simulink model "main_test_all"  (Simulink 6.3)
settings: Solver=ode45  StartTime=0.0  StopTime=6179  RelTol=1e-3
undefined symbols (not defined in the file): A_att_c, B_att_c, C_att_c, D_att_c, ff_on, q_init, q_ref, t_init, t_step
libraries: components_lib x20, simulink x8
settings Model: Creator=krage  LastModifiedBy=mnkr02  ExtModeAutoUpdateStatusClock=off  StrictBusMsg=None
settings DebuggingCC: CheckSSInitialOutputMsg=off

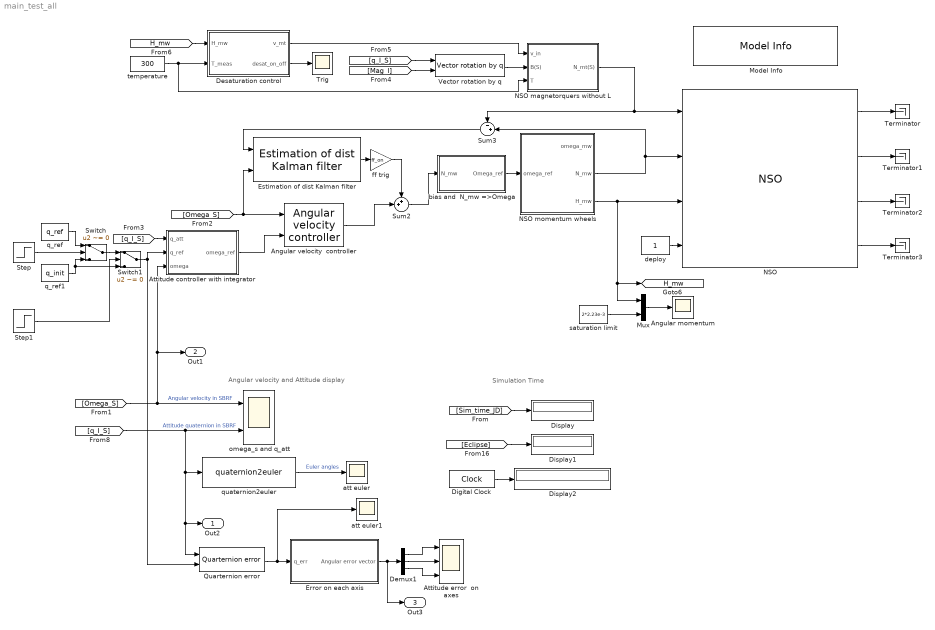
== system main_test_all ==
  note: Simulation Time
  note: Angular velocity and Attitude display
  Angular momentum : Scope
      settings: YMin=0.00125  YMax=0.0045  SaveName=ScopeData2
  Angular velocity  controller : components_lib/ACS/Controllers/Angular velocity  controller  ang_file_name='ang_robust_control.m'
  Attitude controller with integrator : Subsystem  AncestorBlock=components_lib/ACS/Controllers/Attitude controller with integrator  mask(Attitude Controller){att_file_name='att_control_with_integrator.m'}
      mask prompts: att_file_name "Attitude controller design file name (remember gnyfs :-))"
      mask help:
      | The controller in this block is to be constructed using a state space system. The error quarternion is calculated from the input and the result is used in the SS-system. Thus if the controller is merely a gain matrix only the D-matrix has to contain the controller and the remaining be zero-matrices. The controller design files are kept in the "design" directory and the definition of the controller system matrices is the final task in each controller design file.
      | The different matrices for the state space system are named:
      | A_att_c
      | B_att_c
      | C_att_c
      | D_att_c
      mask init:
      | run(strcat('design/',att_file_name))
  Attitude error  on axes : Scope  NumInputPorts=3
      settings: YMin=-3.5~-5~-5  YMax=3.5~5~5  SaveName=ScopeData5
  Demux1 : Demux  Outputs=3
  Desaturation control : Subsystem  mask{h_bias=2.23*1e-3, desat_on=0.7*2.23e-3, desat_off=0.01*2.23e-3}
      mask prompts: h_bias "Angular momentum bias"; desat_on "Threshold desaturation on"; desat_off "Threshold desaturation off"
  Digital Clock : DigitalClock
  Display : Display
  Display1 : Display
  Display2 : Display
  Error on each axis : Subsystem
  Estimation of dist Kalman filter : components_lib/ACS/Controllers/Estimation of dist Kalman filter  ang_file_name='kalman_estimator.m'
  Model Info : simulink/Model-Wide Utilities/Model Info  InitialBlockCM=None  BlockCM=None  Frame=on  DisplayStringWithTags=|  HorizontalTextAlignment=Center  LeftAlignmentValue=0.5  SourceBlockDiagram=main_test_all  TagMaxNumber=20
      | sun to eclipse : 2452315.560376
      | 32 sec. before : 2452315.56
      | eclipse to sun : 2452315.513363
  Mux : Mux  Inputs=2
  NSO : components_lib/NSO  Tag=AAUSAT-II Model  Description=AAUSAT-II Model  r_com_s=[0.05 0.05 0.15]  sat_temp_start=0  r_com_s_deployed=[0.05 0.05 0.125]  mass_sc=3  Dim=[0.1 0.1 0.3]  inertia_c=[25 25 5]/1e3  inertia_d=I_sat  init_jd=2452315.56  q_s_c=[0 0 0 1]  q_init_s_i=q_init  w_init_s=omega_init  Cd=drag_coef  rho=ro_air  enable_sensor_emulation=off  alb_emu_enabled=off  enable_dist=on
  NSO magnetorquers without L : Subsystem  AncestorBlock=components_lib/Actuator Emulation/NSO magnetorquers without L
  NSO momentum wheels : Subsystem  AncestorBlock=components_lib/Actuator Emulation/NSO momentum wheels  mask{w_mw_i=[1078.6 1078.6 1078.6] *0.5}
      mask prompts: w_mw_i "Initial Angular Velocity"
  Quarternion error : components_lib/Math utilities/Quaternion operations/Quarternion error
  Step : Step  Time=t_step  Before=1  After=0  SampleTime=0
  Step1 : Step  Time=t_init  SampleTime=0
  Sum2 : Sum  Inputs=++|
  Sum3 : Sum  Orientation=left  Inputs=-+|
  Switch : Switch  Criteria=u2 ~= 0
  Switch1 : Switch  Criteria=u2 ~= 0
  Terminator{,1..3} (4 alike) : Terminator
  Trig : Scope
      settings: YMin=0.95  YMax=1.05  SaveName=ScopeData3
  Vector rotation by q : components_lib/Math utilities/Quaternion operations/Vector rotation by q
  att euler : Scope
      settings: YMin=-3.5  YMax=3.5
  att euler1 : Scope
      settings: YMin=-3.5  YMax=3.5  SaveName=ScopeData7
  bias and  N_mw =>Omega : Subsystem
  deploy : Constant
  ff trig : Gain  Gain=ff_on
  omega_s and q_att : Scope  NumInputPorts=2
      settings: YMin=-0.4~-1  YMax=0.15~1
  q_ref : Constant  Value=q_ref
  q_ref1 : Constant  Value=q_init
  quaternion2euler : components_lib/Math utilities/Quaternion operations/quaternion2euler
  saturation limit : Constant  Value=2*2.23e-3
  temperature : Constant  Value=300
  Out2 : Outport
  Out1 : Outport  Port=2
  Out3 : Outport  Port=3
  tag scope: H_mw=global
  wires:
  [q_I_S] -> omega_s and q_att/2, quaternion2euler/1, Out2/1, Quarternion error/1  "Attitude quaternion in SBRF"
  quaternion2euler/1 -> att euler/1  "Euler angles"
  [Sim_time_JD] -> Display/1
  [Eclipse] -> Display1/1
  Digital Clock/1 -> Display2/1
  deploy/1 -> NSO/4
  [q_I_S] -> Attitude controller with integrator/1(q_att)
  [Omega_S] -> Angular velocity  controller/1, Estimation of dist Kalman filter/2
  Attitude controller with integrator/1(omega_ref) -> Angular velocity  controller/2
  temperature/1 -> Desaturation control/2(T_meas), NSO magnetorquers without L/3(T)
  [Mag_I] -> Vector rotation by q/2
  [q_I_S] -> Vector rotation by q/1
  Vector rotation by q/1 -> NSO magnetorquers without L/2(B(S))
  Desaturation control/1(v_mt) -> NSO magnetorquers without L/1(v_in)
  [H_mw] -> Desaturation control/1(H_mw)
  NSO magnetorquers without L/1(N_mt(S)) -> NSO/1, Sum3/1
  Desaturation control/2(desat_on_off) -> Trig/1
  NSO momentum wheels/3(H_mw) -> NSO/3, [H_mw], Mux/1
  NSO momentum wheels/2(N_mw) -> NSO/2, Sum3/2
  bias and  N_mw =>Omega/1(Omega_ref) -> NSO momentum wheels/1(omega_ref)
  Mux/1 -> Angular momentum/1
  saturation limit/1 -> Mux/2
  [Omega_S] -> omega_s and q_att/1, Out1/1, Attitude controller with integrator/3(omega)  "Angular velocity in SBRF"
  Angular velocity  controller/1 -> Sum2/2
  Sum2/1 -> bias and  N_mw =>Omega/1(N_mw)
  Sum3/1 -> Estimation of dist Kalman filter/1
  NSO/1 -> Terminator/1
  NSO/2 -> Terminator1/1
  NSO/3 -> Terminator2/1
  NSO/4 -> Terminator3/1
  Estimation of dist Kalman filter/1 -> ff trig/1
  ff trig/1 -> Sum2/1
  Quarternion error/1 -> Error on each axis/1(q_err), att euler1/1
  Error on each axis/1(Angular error vector) -> Demux1/1, Out3/1
  Demux1/1 -> Attitude error  on axes/1
  Demux1/2 -> Attitude error  on axes/2
  Demux1/3 -> Attitude error  on axes/3
  q_ref1/1 -> Switch/3, Switch1/3
  q_ref/1 -> Switch/1
  Step/1 -> Switch/2
  Switch/1 -> Switch1/1
  Switch1/1 -> Attitude controller with integrator/2(q_ref), Quarternion error/2
  Step1/1 -> Switch1/2

== system main_test_all/Attitude controller with integrator ==
  q_att : Inport
  q_ref : Inport  Port=2
  omega : Inport  Port=3
  Integrator : Integrator  LimitOutput=on  UpperSaturationLimit=0.01  LowerSaturationLimit=-0.01
  Mux : Mux  Inputs=3
  Quarternion error : components_lib/Math utilities/Quaternion operations/Quarternion error
  Scope : Scope
      settings: SaveName=ScopeData10
  Selector : Selector  Elements=[1 2 3]  InputPortWidth=4
  State-Space : StateSpace  A=A_att_c  B=B_att_c  C=C_att_c  D=D_att_c
  omega_ref : Outport
  wires:
  Integrator/1 -> Mux/3, Scope/1
  State-Space/1 -> omega_ref/1
  Quarternion error/1 -> Selector/1
  q_att/1 -> Quarternion error/1
  q_ref/1 -> Quarternion error/2
  Selector/1 -> Integrator/1, Mux/1
  omega/1 -> Mux/2
  Mux/1 -> State-Space/1

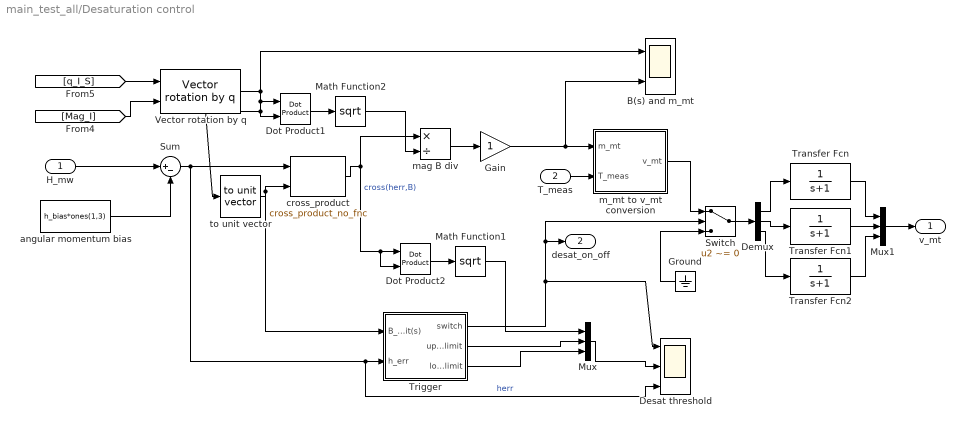
== system main_test_all/Desaturation control ==
  H_mw : Inport
  T_meas : Inport  Port=2
  B(s) and m_mt : Scope  NumInputPorts=2
      settings: YMin=-2e-005~-1  YMax=2e-005~11  SaveName=ScopeData6
  Demux : Demux  Outputs=3
  Desat threshold : Scope  NumInputPorts=3
      settings: YMin=0~0~-0.0025  YMax=1~0.004~0.0025  SaveName=desat_info
  Dot Product1 : simulink/Math Operations/Dot Product  InputSameDT=on  OutDataType=sfix(16)  OutScaling=2^-10  DoSatur=off
  Dot Product2 : simulink/Math Operations/Dot Product  InputSameDT=on  OutDataType=sfix(16)  OutScaling=2^-10  DoSatur=off
  Gain : Gain
  Ground : Ground  Orientation=left
  Math Function1 : Math  Operator=sqrt  SaturateOnIntegerOverflow=on
  Math Function2 : Math  Operator=sqrt  SaturateOnIntegerOverflow=on
  Mux : Mux  Inputs=3
  Mux1 : Mux  Inputs=3
  Sum : Sum  Inputs=|+-
  Switch : Switch  Criteria=u2 ~= 0  Threshold=0.5
  Transfer Fcn : TransferFcn  Denominator=[1 1]
  Transfer Fcn1 : TransferFcn  Denominator=[1 1]
  Transfer Fcn2 : TransferFcn  Denominator=[1 1]
  Trigger : Subsystem
  Vector rotation by q : components_lib/Math utilities/Quaternion operations/Vector rotation by q
  angular momentum bias : Constant  Value=h_bias*ones(1,3)
  cross_product : components_lib/Math utilities/Vector operations/cross_product_no_fnc
  m_mt to v_mt conversion : Subsystem  mask{n_mt=[435 435 865], A_mt=[0.21*0.07 0.21*0.07 0.07*0.07], L_mt=[26.956e-3 26.956e-3 59.256e-3], v_max_mt=5}
      mask prompts: n_mt "Coil winding number [n_x n_y n_z]"; A_mt "Coil area [A_mt_x A_mt_y A_mt_z]"; L_mt "Coil inductance [L_mt_x L_mt_y L_mt_z]"; v_max_mt "Maximum voltage"
  mag B div : Product  Inputs=*/  OutScaling=2^-10
  to unit vector : components_lib/Math utilities/Vector operations/to unit vector
  v_mt : Outport
  desat_on_off : Outport  Port=2
  wires:
  H_mw/1 -> Sum/1
  angular momentum bias/1 -> Sum/2
  [Mag_I] -> Vector rotation by q/2
  [q_I_S] -> Vector rotation by q/1
  Sum/1 -> cross_product/1, Trigger/2(h_err), Desat threshold/3  "herr"
  Vector rotation by q/1 -> Dot Product1/1, Dot Product1/2, to unit vector/1, B(s) and m_mt/1
  cross_product/1 -> mag B div/1, Dot Product2/1, Dot Product2/2  "cross(herr,B)"
  Ground/1 -> Switch/3
  T_meas/1 -> m_mt to v_mt conversion/2(T_meas)
  mag B div/1 -> Gain/1
  m_mt to v_mt conversion/1(v_mt) -> Switch/1
  Dot Product1/1 -> Math Function2/1
  Math Function2/1 -> mag B div/2
  Gain/1 -> m_mt to v_mt conversion/1(m_mt), B(s) and m_mt/2
  to unit vector/1 -> cross_product/2, Trigger/1(B_unit(s))
  Switch/1 -> Demux/1
  Demux/1 -> Transfer Fcn/1
  Demux/2 -> Transfer Fcn1/1
  Demux/3 -> Transfer Fcn2/1
  Transfer Fcn/1 -> Mux1/1
  Transfer Fcn1/1 -> Mux1/2
  Transfer Fcn2/1 -> Mux1/3
  Mux1/1 -> v_mt/1
  Mux/1 -> Desat threshold/2
  Trigger/1(switch) -> Desat threshold/1, desat_on_off/1, Switch/2
  Trigger/2(upper limit) -> Mux/2
  Dot Product2/1 -> Math Function1/1
  Math Function1/1 -> Mux/1
  Trigger/3(lower limit) -> Mux/3

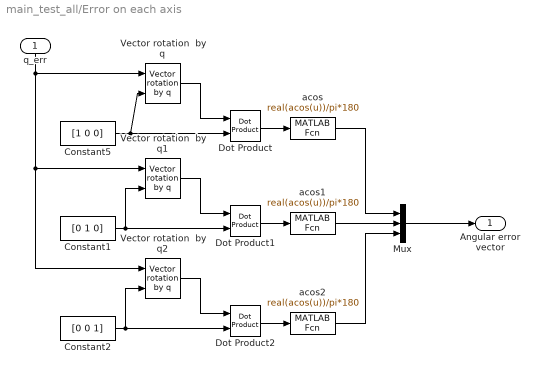
== system main_test_all/Error on each axis ==
  q_err : Inport  Orientation=down
  Constant1 : Constant  Value=[0 1 0]
  Constant2 : Constant  Value=[0 0 1]
  Constant5 : Constant  Value=[1 0 0]
  Dot Product : simulink/Math Operations/Dot Product  InputSameDT=on  OutDataType=sfix(16)  OutScaling=2^-10  DoSatur=off
  Dot Product1 : simulink/Math Operations/Dot Product  InputSameDT=on  OutDataType=sfix(16)  OutScaling=2^-10  DoSatur=off
  Dot Product2 : simulink/Math Operations/Dot Product  InputSameDT=on  OutDataType=sfix(16)  OutScaling=2^-10  DoSatur=off
  Mux : Mux  Inputs=3
  Vector rotation  by q : components_lib/Math utilities/Quaternion operations/Vector rotation by q
  Vector rotation  by q1 : components_lib/Math utilities/Quaternion operations/Vector rotation by q
  Vector rotation  by q2 : components_lib/Math utilities/Quaternion operations/Vector rotation by q
  acos : MATLABFcn  MATLABFcn=real(acos(u))/pi*180
  acos1 : MATLABFcn  MATLABFcn=real(acos(u))/pi*180
  acos2 : MATLABFcn  MATLABFcn=real(acos(u))/pi*180
  Angular error vector : Outport
  wires:
  Constant5/1 -> Dot Product/2, Vector rotation  by q/2
  Vector rotation  by q/1 -> Dot Product/1
  Dot Product/1 -> acos/1
  q_err/1 -> Vector rotation  by q/1, Vector rotation  by q1/1, Vector rotation  by q2/1
  Constant1/1 -> Vector rotation  by q1/2, Dot Product1/2
  Vector rotation  by q1/1 -> Dot Product1/1
  Dot Product1/1 -> acos1/1
  Constant2/1 -> Vector rotation  by q2/2, Dot Product2/2
  Vector rotation  by q2/1 -> Dot Product2/1
  Dot Product2/1 -> acos2/1
  acos/1 -> Mux/1
  acos1/1 -> Mux/2
  acos2/1 -> Mux/3
  Mux/1 -> Angular error vector/1

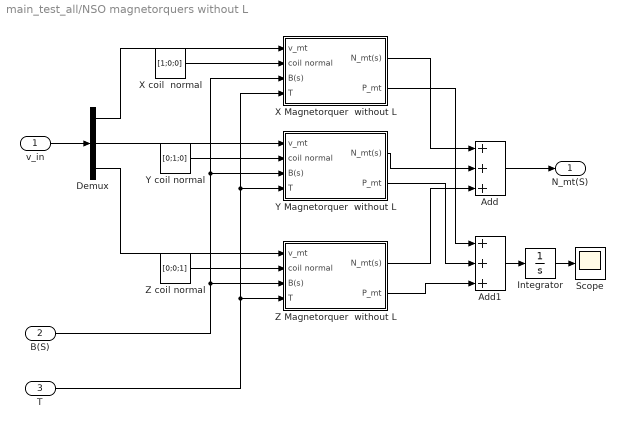
== system main_test_all/NSO magnetorquers without L ==
  v_in : Inport
  B(S) : Inport  Port=2
  T : Inport  Port=3
  Add : Sum  Inputs=+++  OutScaling=2^-10
  Add1 : Sum  Inputs=+++  OutScaling=2^-10
  Demux : Demux  Outputs=3
  Integrator : Integrator
  Scope : Scope
      settings: YMin=24.35  YMax=25.2  SaveName=power_mt
  "X Magnetorquer  without L " : Subsystem  AncestorBlock=components_lib/Actuator Emulation/Magnetorquer without L  mask{v_max_mt=5, coil_dim=[0.07 0.21], n_mt=435, A_wire_mt=(pi/4)*0.0002^2, sigma_0_mt=1.7e-8, alpha_0_mt=3.9e-3, T_0_mt=293}
      mask prompts: v_max_mt "Maximum voltage"; coil_dim "Coil dimensions [x y]"; n_mt "Coil winding number"; A_wire_mt "Wire cross sectional area"; sigma_0_mt "Wire resistivity"; alpha_0_mt "Wire resistivity temp. coef."; T_0_mt "Wire resistivity base temp."
  X coil  normal : Constant  Value=[1;0;0]
  Y Magnetorquer  without L : Subsystem  AncestorBlock=components_lib/Actuator Emulation/Magnetorquer without L  mask{v_max_mt=5, coil_dim=[0.07 0.21], n_mt=435, A_wire_mt=(pi/4)*0.0002^2, sigma_0_mt=1.7e-8, alpha_0_mt=3.9e-3, T_0_mt=293}
      mask prompts: v_max_mt "Maximum voltage"; coil_dim "Coil dimensions [x y]"; n_mt "Coil winding number"; A_wire_mt "Wire cross sectional area"; sigma_0_mt "Wire resistivity"; alpha_0_mt "Wire resistivity temp. coef."; T_0_mt "Wire resistivity base temp."
  Y coil normal : Constant  Value=[0;1;0]
  Z Magnetorquer  without L : Subsystem  AncestorBlock=components_lib/Actuator Emulation/Magnetorquer without L  mask{v_max_mt=5, coil_dim=[0.07 0.07], n_mt=865, A_wire_mt=(pi/4)*0.0002^2, sigma_0_mt=1.7e-8, alpha_0_mt=3.9e-3, T_0_mt=293}
      mask prompts: v_max_mt "Maximum voltage"; coil_dim "Coil dimensions [x y]"; n_mt "Coil winding number"; A_wire_mt "Wire cross sectional area"; sigma_0_mt "Wire resistivity"; alpha_0_mt "Wire resistivity temp. coef."; T_0_mt "Wire resistivity base temp."
  Z coil normal : Constant  Value=[0;0;1]
  N_mt(S) : Outport  PortDimensions=3
  wires:
  v_in/1 -> Demux/1
  Add/1 -> N_mt(S)/1
  X coil  normal/1 -> "X Magnetorquer  without L "/2(coil normal)
  Demux/1 -> "X Magnetorquer  without L "/1(v_mt)
  "X Magnetorquer  without L "/1(N_mt(s)) -> Add/1
  Y Magnetorquer  without L/1(N_mt(s)) -> Add/2
  Z Magnetorquer  without L/1(N_mt(s)) -> Add/3
  Demux/2 -> Y Magnetorquer  without L/1(v_mt)
  Y coil normal/1 -> Y Magnetorquer  without L/2(coil normal)
  Demux/3 -> Z Magnetorquer  without L/1(v_mt)
  Z coil normal/1 -> Z Magnetorquer  without L/2(coil normal)
  B(S)/1 -> Z Magnetorquer  without L/3(B(s)), Y Magnetorquer  without L/3(B(s)), "X Magnetorquer  without L "/3(B(s))
  T/1 -> Z Magnetorquer  without L/4(T), Y Magnetorquer  without L/4(T), "X Magnetorquer  without L "/4(T)
  "X Magnetorquer  without L "/2(P_mt) -> Add1/1
  Y Magnetorquer  without L/2(P_mt) -> Add1/2
  Z Magnetorquer  without L/2(P_mt) -> Add1/3
  Add1/1 -> Integrator/1
  Integrator/1 -> Scope/1

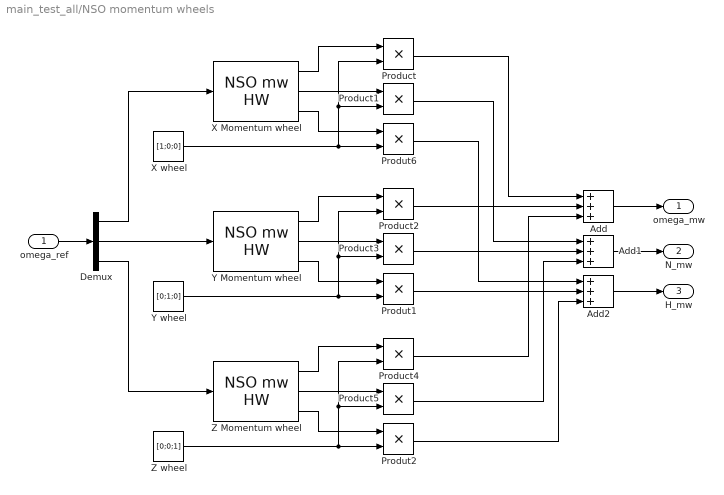
== system main_test_all/NSO momentum wheels ==
  omega_ref : Inport
  Add : Sum  Inputs=+++  OutScaling=2^-10
  Add1 : Sum  Inputs=+++  OutScaling=2^-10
  Add2 : Sum  Inputs=+++  OutScaling=2^-10
  Demux : Demux  Outputs=3
  Product{,1..5} (6 alike) : Product  RndMeth=Zero
  Produt1 : Product  RndMeth=Zero
  Produt2 : Product  RndMeth=Zero
  Produt6 : Product  RndMeth=Zero
  X Momentum wheel : components_lib/Actuator Emulation/NSO mw HW  C_p=0.01  C_i=0.001  w_mw_init=w_mw_i(1)
  X wheel : Constant  Value=[1;0;0]
  Y Momentum wheel : components_lib/Actuator Emulation/NSO mw HW  C_p=0.01  C_i=0.001  w_mw_init=w_mw_i(2)
  Y wheel : Constant  Value=[0;1;0]
  Z Momentum wheel : components_lib/Actuator Emulation/NSO mw HW  C_p=0.01  C_i=0.001  w_mw_init=w_mw_i(3)
  Z wheel : Constant  Value=[0;0;1]
  omega_mw : Outport  PortDimensions=3
  N_mw : Outport  Port=2  PortDimensions=3
  H_mw : Outport  Port=3  PortDimensions=3
  wires:
  Demux/2 -> Y Momentum wheel/1
  Demux/3 -> Z Momentum wheel/1
  Demux/1 -> X Momentum wheel/1
  omega_ref/1 -> Demux/1
  Product4/1 -> Add/3
  Product5/1 -> Add1/3
  Produt2/1 -> Add2/3
  Z Momentum wheel/2 -> Product5/1
  Z Momentum wheel/1 -> Product4/1
  Z Momentum wheel/3 -> Produt2/1
  Z wheel/1 -> Produt2/2, Product5/2, Product4/2
  Produt1/1 -> Add2/2
  Product3/1 -> Add1/2
  Product2/1 -> Add/2
  Y Momentum wheel/2 -> Product3/1
  Y Momentum wheel/1 -> Product2/1
  Y Momentum wheel/3 -> Produt1/1
  Y wheel/1 -> Produt1/2, Product3/2, Product2/2
  X Momentum wheel/2 -> Product1/1
  X Momentum wheel/1 -> Product/1
  X Momentum wheel/3 -> Produt6/1
  Add/1 -> omega_mw/1
  X wheel/1 -> Produt6/2, Product1/2, Product/2
  Add1/1 -> N_mw/1
  Product/1 -> Add/1
  Product1/1 -> Add1/1
  Add2/1 -> H_mw/1
  Produt6/1 -> Add2/1

== system main_test_all/bias and  N_mw =>Omega ==
  N_mw : Inport
  I_FW : Gain  Gain=1/4.139e-6
  Integrator : Integrator  InitialCondition=[2.23 2.23 2.23]*1e-3
  Sum : Sum  Inputs=|++
  angular velocity bias : Constant  Value=[1078.6 1078.6 1078.6] *0.5
  Omega_ref : Outport
  wires:
  I_FW/1 -> Sum/1
  angular velocity bias/1 -> Sum/2
  Integrator/1 -> I_FW/1
  N_mw/1 -> Integrator/1
  Sum/1 -> Omega_ref/1

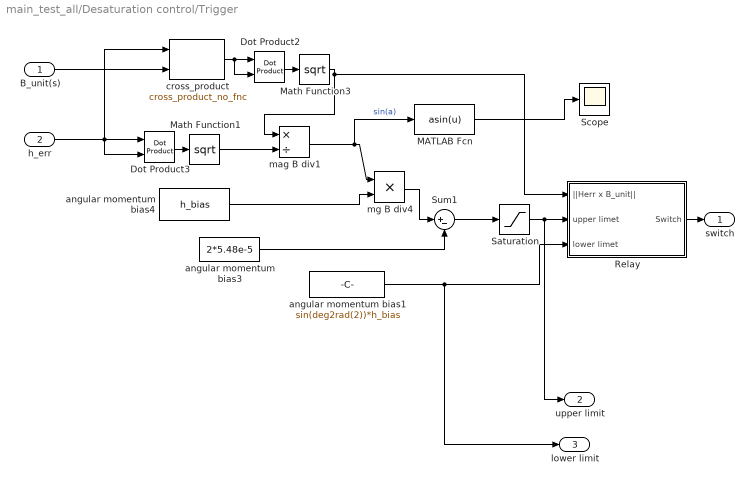
== system main_test_all/Desaturation control/Trigger ==
  B_unit(s) : Inport  PortDimensions=3
  h_err : Inport  Port=2
  Dot Product2 : simulink/Math Operations/Dot Product  InputSameDT=on  OutDataType=sfix(16)  OutScaling=2^-10  DoSatur=off
  Dot Product3 : simulink/Math Operations/Dot Product  InputSameDT=on  OutDataType=sfix(16)  OutScaling=2^-10  DoSatur=off
  MATLAB Fcn : MATLABFcn  MATLABFcn=asin(u)
  Math Function1 : Math  Operator=sqrt  SaturateOnIntegerOverflow=on
  Math Function3 : Math  Operator=sqrt  SaturateOnIntegerOverflow=on
  Relay : Subsystem
  Saturation : Saturate  UpperLimit=inf  LowerLimit=2*sin(deg2rad(2))*h_bias
  Scope : Scope
      settings: YMin=0.5  YMax=1.6  SaveName=ScopeData4
  Sum1 : Sum  Inputs=|+-
  angular momentum bias1 : Constant  Value=sin(deg2rad(2))*h_bias
  angular momentum bias3 : Constant  Value=2*5.48e-5
  angular momentum bias4 : Constant  Value=h_bias
  cross_product : components_lib/Math utilities/Vector operations/cross_product_no_fnc
  mag B div1 : Product  Inputs=*/  OutScaling=2^-10
  mg B div4 : Product  OutScaling=2^-10
  switch : Outport
  upper limit : Outport  Port=2
  lower limit : Outport  Port=3
  wires:
  angular momentum bias3/1 -> Sum1/2
  Relay/1(Switch) -> switch/1
  angular momentum bias4/1 -> mg B div4/2
  mg B div4/1 -> Sum1/1
  Dot Product2/1 -> Math Function3/1
  Dot Product3/1 -> Math Function1/1
  Math Function1/1 -> mag B div1/2
  Sum1/1 -> Saturation/1
  mag B div1/1 -> mg B div4/1, MATLAB Fcn/1  "sin(a)"
  h_err/1 -> Dot Product3/1, Dot Product3/2, cross_product/1
  B_unit(s)/1 -> cross_product/2
  cross_product/1 -> Dot Product2/1, Dot Product2/2
  Math Function3/1 -> mag B div1/1, Relay/1(||Herr x B_unit||)
  angular momentum bias1/1 -> Relay/3(lower limet), lower limit/1
  MATLAB Fcn/1 -> Scope/1
  Saturation/1 -> Relay/2(upper limet), upper limit/1

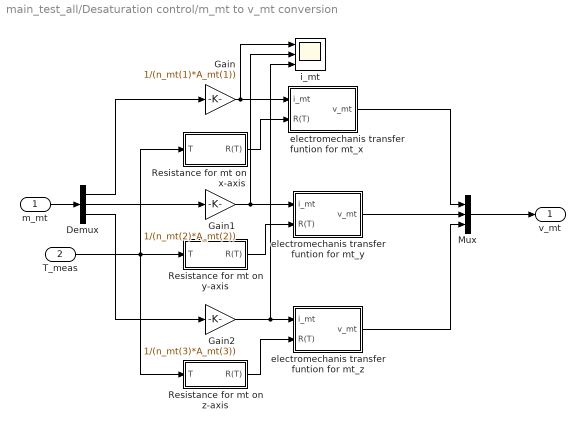
== system main_test_all/Desaturation control/m_mt to v_mt conversion ==
  m_mt : Inport
  T_meas : Inport  Port=2
  Demux : Demux  Outputs=3
  Gain : Gain  Gain=1/(n_mt(1)*A_mt(1))
  Gain1 : Gain  Gain=1/(n_mt(2)*A_mt(2))
  Gain2 : Gain  Gain=1/(n_mt(3)*A_mt(3))
  Mux : Mux  Inputs=3
  Resistance for mt on x-axis : Subsystem  mask{A_wire_mt=(pi/4)*0.0002^2, sigma_0_mt=1.7e-8, alpha_0_mt=3.9e-3, T_0_mt=293}
      mask prompts: A_wire_mt "Wire cross sectional area"; sigma_0_mt "Wire resistivity"; alpha_0_mt "Wire resistivity temp. coef."; T_0_mt "Wire resistivity base temp."
  Resistance for mt on y-axis : Subsystem  mask{A_wire_mt=(pi/4)*0.0002^2, sigma_0_mt=1.7e-8, alpha_0_mt=3.9e-3, T_0_mt=293}
      mask prompts: A_wire_mt "Wire cross sectional area"; sigma_0_mt "Wire resistivity"; alpha_0_mt "Wire resistivity temp. coef."; T_0_mt "Wire resistivity base temp."
  Resistance for mt on z-axis : Subsystem  mask{A_wire_mt=(pi/4)*0.0002^2, sigma_0_mt=1.7e-8, alpha_0_mt=3.9e-3, T_0_mt=293}
      mask prompts: A_wire_mt "Wire cross sectional area"; sigma_0_mt "Wire resistivity"; alpha_0_mt "Wire resistivity temp. coef."; T_0_mt "Wire resistivity base temp."
  electromechanis transfer funtion for mt_x : Subsystem
  "electromechanis transfer funtion for mt_y " : Subsystem
  "electromechanis transfer funtion for mt_z " : Subsystem
  i_mt : Scope  NumInputPorts=3
      settings: YMin=-5~-5~-5  YMax=5~5~5  SaveName=ScopeData8
  v_mt : Outport
  wires:
  Demux/3 -> Gain2/1
  Demux/2 -> Gain1/1
  Demux/1 -> Gain/1
  Gain/1 -> electromechanis transfer funtion for mt_x/1(i_mt), i_mt/1
  Gain1/1 -> "electromechanis transfer funtion for mt_y "/1(i_mt), i_mt/2
  Gain2/1 -> "electromechanis transfer funtion for mt_z "/1(i_mt), i_mt/3
  m_mt/1 -> Demux/1
  "electromechanis transfer funtion for mt_y "/1(v_mt) -> Mux/2
  "electromechanis transfer funtion for mt_z "/1(v_mt) -> Mux/3
  Resistance for mt on x-axis/1(R(T)) -> electromechanis transfer funtion for mt_x/2(R(T))
  Resistance for mt on y-axis/1(R(T)) -> "electromechanis transfer funtion for mt_y "/2(R(T))
  Resistance for mt on z-axis/1(R(T)) -> "electromechanis transfer funtion for mt_z "/2(R(T))
  T_meas/1 -> Resistance for mt on y-axis/1(T), Resistance for mt on x-axis/1(T), Resistance for mt on z-axis/1(T)
  electromechanis transfer funtion for mt_x/1(v_mt) -> Mux/1
  Mux/1 -> v_mt/1

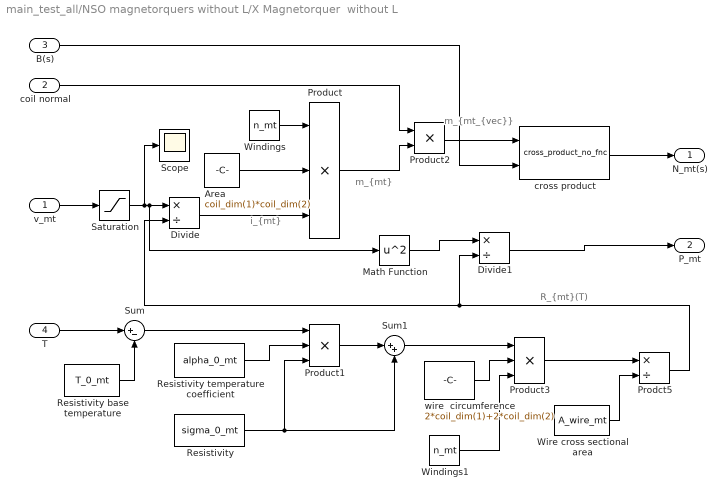
== system main_test_all/NSO magnetorquers without L/X Magnetorquer  without L  ==
  note: R_{mt}(T)
  note: i_{mt}
  note: m_{mt}
  note: m_{mt_{vec}}
  v_mt : Inport
  coil normal : Inport  Port=2
  B(s) : Inport  Port=3
  T : Inport  Port=4
  Area : Constant  Value=coil_dim(1)*coil_dim(2)
  Divide : Product  Inputs=*/  OutScaling=2^-10
  Divide1 : Product  Inputs=*/  OutScaling=2^-10
  Math Function : Math  Operator=square  SaturateOnIntegerOverflow=on
  Prodct5 : Product  Inputs=*/  RndMeth=Zero
  Product : Product  Inputs=3  RndMeth=Zero
  Product1 : Product  Inputs=3  RndMeth=Zero
  Product2 : Product  RndMeth=Zero
  Product3 : Product  Inputs=3  RndMeth=Zero
  Resistivity : Constant  Value=sigma_0_mt
  Resistivity base temperature : Constant  Value=T_0_mt
  Resistivity temperature coefficient : Constant  Value=alpha_0_mt
  Saturation : Saturate  UpperLimit=v_max_mt  LowerLimit=-v_max_mt
  Scope : Scope
      settings: SaveName=ScopeData12
  Sum : Sum  Inputs=|+-
  Sum1 : Sum  Inputs=|++
  Windings : Constant  Value=n_mt
  Windings1 : Constant  Value=n_mt
  Wire cross sectional area : Constant  Value=A_wire_mt
  cross product : components_lib/Math utilities/Vector operations/cross_product_no_fnc
  wire  circumference : Constant  Value=2*coil_dim(1)+2*coil_dim(2)
  N_mt(s) : Outport
  P_mt : Outport  Port=2
  wires:
  Prodct5/1 -> Divide/2, Divide1/2
  Wire cross sectional area/1 -> Prodct5/2
  Product3/1 -> Prodct5/1
  Windings1/1 -> Product3/3
  wire  circumference/1 -> Product3/2
  Sum1/1 -> Product3/1
  Product1/1 -> Sum1/1
  Resistivity/1 -> Sum1/2, Product1/3
  Sum/1 -> Product1/1
  Resistivity temperature coefficient/1 -> Product1/2
  T/1 -> Sum/1
  Resistivity base temperature/1 -> Sum/2
  coil normal/1 -> Product2/1
  v_mt/1 -> Saturation/1
  Saturation/1 -> Divide/1, Math Function/1, Scope/1
  Divide/1 -> Product/3
  Windings/1 -> Product/1
  Area/1 -> Product/2
  Product/1 -> Product2/2
  Product2/1 -> cross product/1
  cross product/1 -> N_mt(s)/1
  B(s)/1 -> cross product/2
  Math Function/1 -> Divide1/1
  Divide1/1 -> P_mt/1

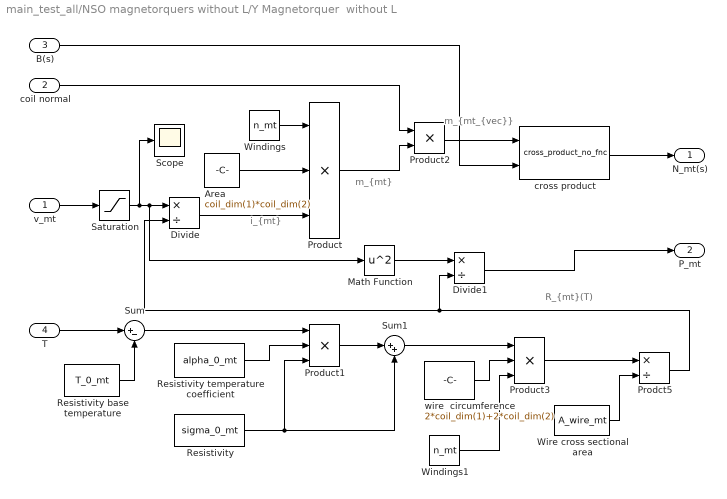
== system main_test_all/NSO magnetorquers without L/Y Magnetorquer  without L ==
  note: R_{mt}(T)
  note: i_{mt}
  note: m_{mt}
  note: m_{mt_{vec}}
  v_mt : Inport
  coil normal : Inport  Port=2
  B(s) : Inport  Port=3
  T : Inport  Port=4
  Area : Constant  Value=coil_dim(1)*coil_dim(2)
  Divide : Product  Inputs=*/  OutScaling=2^-10
  Divide1 : Product  Inputs=*/  OutScaling=2^-10
  Math Function : Math  Operator=square  SaturateOnIntegerOverflow=on
  Prodct5 : Product  Inputs=*/  RndMeth=Zero
  Product : Product  Inputs=3  RndMeth=Zero
  Product1 : Product  Inputs=3  RndMeth=Zero
  Product2 : Product  RndMeth=Zero
  Product3 : Product  Inputs=3  RndMeth=Zero
  Resistivity : Constant  Value=sigma_0_mt
  Resistivity base temperature : Constant  Value=T_0_mt
  Resistivity temperature coefficient : Constant  Value=alpha_0_mt
  Saturation : Saturate  UpperLimit=v_max_mt  LowerLimit=-v_max_mt
  Scope : Scope
      settings: SaveName=ScopeData13
  Sum : Sum  Inputs=|+-
  Sum1 : Sum  Inputs=|++
  Windings : Constant  Value=n_mt
  Windings1 : Constant  Value=n_mt
  Wire cross sectional area : Constant  Value=A_wire_mt
  cross product : components_lib/Math utilities/Vector operations/cross_product_no_fnc
  wire  circumference : Constant  Value=2*coil_dim(1)+2*coil_dim(2)
  N_mt(s) : Outport
  P_mt : Outport  Port=2
  wires:
  Prodct5/1 -> Divide/2, Divide1/2
  Wire cross sectional area/1 -> Prodct5/2
  Product3/1 -> Prodct5/1
  Windings1/1 -> Product3/3
  wire  circumference/1 -> Product3/2
  Sum1/1 -> Product3/1
  Product1/1 -> Sum1/1
  Resistivity/1 -> Sum1/2, Product1/3
  Sum/1 -> Product1/1
  Resistivity temperature coefficient/1 -> Product1/2
  T/1 -> Sum/1
  Resistivity base temperature/1 -> Sum/2
  coil normal/1 -> Product2/1
  v_mt/1 -> Saturation/1
  Saturation/1 -> Divide/1, Math Function/1, Scope/1
  Divide/1 -> Product/3
  Windings/1 -> Product/1
  Area/1 -> Product/2
  Product/1 -> Product2/2
  Product2/1 -> cross product/1
  cross product/1 -> N_mt(s)/1
  B(s)/1 -> cross product/2
  Math Function/1 -> Divide1/1
  Divide1/1 -> P_mt/1

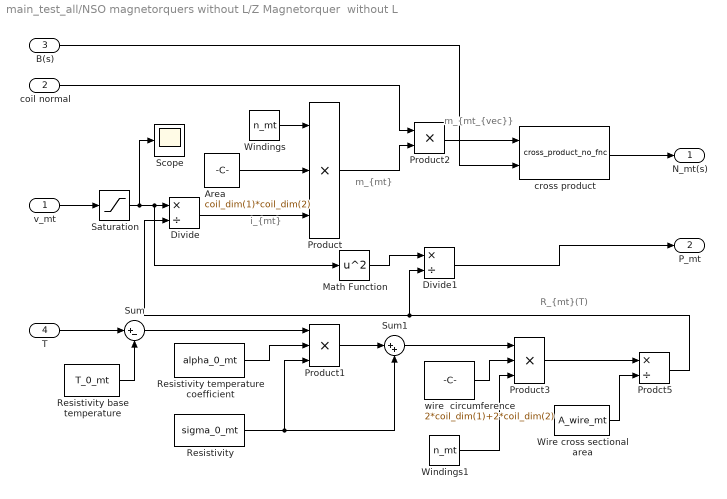
== system main_test_all/NSO magnetorquers without L/Z Magnetorquer  without L ==
  note: R_{mt}(T)
  note: i_{mt}
  note: m_{mt}
  note: m_{mt_{vec}}
  v_mt : Inport
  coil normal : Inport  Port=2
  B(s) : Inport  Port=3
  T : Inport  Port=4
  Area : Constant  Value=coil_dim(1)*coil_dim(2)
  Divide : Product  Inputs=*/  OutScaling=2^-10
  Divide1 : Product  Inputs=*/  OutScaling=2^-10
  Math Function : Math  Operator=square  SaturateOnIntegerOverflow=on
  Prodct5 : Product  Inputs=*/  RndMeth=Zero
  Product : Product  Inputs=3  RndMeth=Zero
  Product1 : Product  Inputs=3  RndMeth=Zero
  Product2 : Product  RndMeth=Zero
  Product3 : Product  Inputs=3  RndMeth=Zero
  Resistivity : Constant  Value=sigma_0_mt
  Resistivity base temperature : Constant  Value=T_0_mt
  Resistivity temperature coefficient : Constant  Value=alpha_0_mt
  Saturation : Saturate  UpperLimit=v_max_mt  LowerLimit=-v_max_mt
  Scope : Scope
      settings: YMin=-1.5  SaveName=ScopeData14
  Sum : Sum  Inputs=|+-
  Sum1 : Sum  Inputs=|++
  Windings : Constant  Value=n_mt
  Windings1 : Constant  Value=n_mt
  Wire cross sectional area : Constant  Value=A_wire_mt
  cross product : components_lib/Math utilities/Vector operations/cross_product_no_fnc
  wire  circumference : Constant  Value=2*coil_dim(1)+2*coil_dim(2)
  N_mt(s) : Outport
  P_mt : Outport  Port=2
  wires:
  Prodct5/1 -> Divide/2, Divide1/2
  Wire cross sectional area/1 -> Prodct5/2
  Product3/1 -> Prodct5/1
  Windings1/1 -> Product3/3
  wire  circumference/1 -> Product3/2
  Sum1/1 -> Product3/1
  Product1/1 -> Sum1/1
  Resistivity/1 -> Sum1/2, Product1/3
  Sum/1 -> Product1/1
  Resistivity temperature coefficient/1 -> Product1/2
  T/1 -> Sum/1
  Resistivity base temperature/1 -> Sum/2
  coil normal/1 -> Product2/1
  v_mt/1 -> Saturation/1
  Saturation/1 -> Divide/1, Math Function/1, Scope/1
  Divide/1 -> Product/3
  Windings/1 -> Product/1
  Area/1 -> Product/2
  Product/1 -> Product2/2
  Product2/1 -> cross product/1
  cross product/1 -> N_mt(s)/1
  B(s)/1 -> cross product/2
  Math Function/1 -> Divide1/1
  Divide1/1 -> P_mt/1

== system main_test_all/Desaturation control/Trigger/Relay ==
  ||Herr x B_unit|| : Inport  Orientation=down
  upper limet : Inport  Port=2
  lower limet : Inport  Port=3
  Logical Operator1 : Logic  AllPortsSameDT=off  OutDataTypeMode=Boolean
  Logical Operator2 : Logic  Operator=OR  AllPortsSameDT=off  OutDataTypeMode=Boolean
  Logical Operator3 : Logic  AllPortsSameDT=off  OutDataTypeMode=Boolean
  Memory : Memory  Orientation=left
  Relational Operator : RelationalOperator  Operator=>  LogicOutDataTypeMode=Boolean  LogicDataType=1
  Relational Operator1 : RelationalOperator  Operator=>  LogicOutDataTypeMode=Boolean  LogicDataType=1
  Switch : Outport
  wires:
  ||Herr x B_unit||/1 -> Relational Operator/1, Relational Operator1/1
  Relational Operator1/1 -> Logical Operator1/1, Logical Operator3/2
  Logical Operator1/1 -> Logical Operator2/2
  Logical Operator2/1 -> Memory/1, Switch/1
  Memory/1 -> Logical Operator1/2
  upper limet/1 -> Relational Operator/2
  lower limet/1 -> Relational Operator1/2
  Relational Operator/1 -> Logical Operator3/1
  Logical Operator3/1 -> Logical Operator2/1

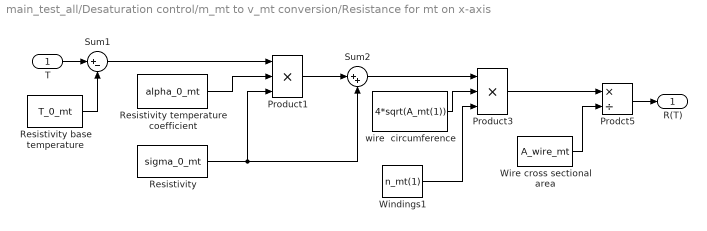
== system main_test_all/Desaturation control/m_mt to v_mt conversion/Resistance for mt on x-axis ==
  T : Inport
  Prodct5 : Product  Inputs=*/  RndMeth=Zero
  Product1 : Product  Inputs=3  RndMeth=Zero
  Product3 : Product  Inputs=3  RndMeth=Zero
  Resistivity : Constant  Value=sigma_0_mt
  Resistivity base temperature : Constant  Value=T_0_mt
  Resistivity temperature coefficient : Constant  Value=alpha_0_mt
  Sum1 : Sum  Inputs=|+-
  Sum2 : Sum  Inputs=|++
  Windings1 : Constant  Value=n_mt(1)
  Wire cross sectional area : Constant  Value=A_wire_mt
  wire  circumference : Constant  Value=4*sqrt(A_mt(1))
  R(T) : Outport
  wires:
  Resistivity base temperature/1 -> Sum1/2
  Resistivity temperature coefficient/1 -> Product1/2
  Sum1/1 -> Product1/1
  Resistivity/1 -> Product1/3, Sum2/2
  Product1/1 -> Sum2/1
  Sum2/1 -> Product3/1
  wire  circumference/1 -> Product3/2
  Windings1/1 -> Product3/3
  Product3/1 -> Prodct5/1
  Wire cross sectional area/1 -> Prodct5/2
  T/1 -> Sum1/1
  Prodct5/1 -> R(T)/1

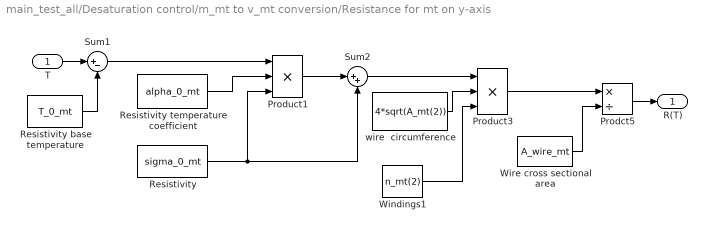
== system main_test_all/Desaturation control/m_mt to v_mt conversion/Resistance for mt on y-axis ==
  T : Inport
  Prodct5 : Product  Inputs=*/  RndMeth=Zero
  Product1 : Product  Inputs=3  RndMeth=Zero
  Product3 : Product  Inputs=3  RndMeth=Zero
  Resistivity : Constant  Value=sigma_0_mt
  Resistivity base temperature : Constant  Value=T_0_mt
  Resistivity temperature coefficient : Constant  Value=alpha_0_mt
  Sum1 : Sum  Inputs=|+-
  Sum2 : Sum  Inputs=|++
  Windings1 : Constant  Value=n_mt(2)
  Wire cross sectional area : Constant  Value=A_wire_mt
  wire  circumference : Constant  Value=4*sqrt(A_mt(2))
  R(T) : Outport
  wires:
  Prodct5/1 -> R(T)/1
  T/1 -> Sum1/1
  Wire cross sectional area/1 -> Prodct5/2
  Product3/1 -> Prodct5/1
  Windings1/1 -> Product3/3
  wire  circumference/1 -> Product3/2
  Sum2/1 -> Product3/1
  Product1/1 -> Sum2/1
  Resistivity/1 -> Sum2/2, Product1/3
  Sum1/1 -> Product1/1
  Resistivity temperature coefficient/1 -> Product1/2
  Resistivity base temperature/1 -> Sum1/2

== system main_test_all/Desaturation control/m_mt to v_mt conversion/Resistance for mt on z-axis ==
  T : Inport
  Prodct5 : Product  Inputs=*/  RndMeth=Zero
  Product1 : Product  Inputs=3  RndMeth=Zero
  Product3 : Product  Inputs=3  RndMeth=Zero
  Resistivity : Constant  Value=sigma_0_mt
  Resistivity base temperature : Constant  Value=T_0_mt
  Resistivity temperature coefficient : Constant  Value=alpha_0_mt
  Sum1 : Sum  Inputs=|+-
  Sum2 : Sum  Inputs=|++
  Windings1 : Constant  Value=n_mt(3)
  Wire cross sectional area : Constant  Value=A_wire_mt
  wire  circumference : Constant  Value=4*sqrt(A_mt(3))
  R(T) : Outport
  wires:
  Resistivity base temperature/1 -> Sum1/2
  Resistivity temperature coefficient/1 -> Product1/2
  Sum1/1 -> Product1/1
  Resistivity/1 -> Product1/3, Sum2/2
  Product1/1 -> Sum2/1
  Sum2/1 -> Product3/1
  wire  circumference/1 -> Product3/2
  Windings1/1 -> Product3/3
  Product3/1 -> Prodct5/1
  Wire cross sectional area/1 -> Prodct5/2
  T/1 -> Sum1/1
  Prodct5/1 -> R(T)/1

== system main_test_all/Desaturation control/m_mt to v_mt conversion/electromechanis transfer funtion for mt_x ==
  i_mt : Inport
  R(T) : Inport  Port=2
  Derivative : Derivative
  Gain : Gain  Gain=L_mt(1)
  Product1 : Product  RndMeth=Zero
  Scope : Scope  NumInputPorts=3
      settings: YMin=-5~-5~-5  YMax=5~5~5  SaveName=ScopeData9
  Sum : Sum  Inputs=++|
  v_mt : Outport
  wires:
  Derivative/1 -> Gain/1, Scope/1
  Sum/1 -> v_mt/1, Scope/3
  i_mt/1 -> Derivative/1, Product1/1
  R(T)/1 -> Product1/2, Scope/2
  Product1/1 -> Sum/2
  Gain/1 -> Sum/1

== system main_test_all/Desaturation control/m_mt to v_mt conversion/electromechanis transfer funtion for mt_y  ==
  i_mt : Inport
  R(T) : Inport  Port=2
  Derivative : Derivative
  Gain : Gain  Gain=L_mt(2)
  Product1 : Product  RndMeth=Zero
  Sum : Sum  Inputs=++|
  v_mt : Outport
  wires:
  Gain/1 -> Sum/1
  Product1/1 -> Sum/2
  R(T)/1 -> Product1/2
  i_mt/1 -> Product1/1, Derivative/1
  Sum/1 -> v_mt/1
  Derivative/1 -> Gain/1

== system main_test_all/Desaturation control/m_mt to v_mt conversion/electromechanis transfer funtion for mt_z  ==
  i_mt : Inport
  R(T) : Inport  Port=2
  Derivative : Derivative
  Gain : Gain  Gain=L_mt(3)
  Product1 : Product  RndMeth=Zero
  Sum : Sum  Inputs=++|
  v_mt : Outport
  wires:
  Derivative/1 -> Gain/1
  Sum/1 -> v_mt/1
  i_mt/1 -> Derivative/1, Product1/1
  R(T)/1 -> Product1/2
  Product1/1 -> Sum/2
  Gain/1 -> Sum/1
